simulink model "Test_Model_HR12_2016"  (R2016b)
settings: Solver=FixedStepAuto  StartTime=0.0  StopTime=length(ipoint)  FixedStep=dt  RelTol=1e-3
values from neighbouring files (symbols this model uses):
  Cbx_cyl_fill_efy_intk_mfld_prs_atm_prs_cor_cho = true    [Calib_mdl_RSA.m]
  Cbx_cyl_fill_efy_opt_cho = false    [Calib_mdl_RSA.m]
  Cbx_cyl_fill_igr_opt_cho = false    [Calib_mdl_RSA.m]
  Cbx_ex_vvt_conf = true    [Calib_mdl_RSA.m]
  Cnx_cyl_fill_ex_mfld_prs_cor_cho = 0    [Cal_basic.m]
  Cnx_cyl_nr_conf = 3    [Cal_basic.m]
  Cxx_cyl_fill_efy_drv_max = 20    [Calib_mdl_RSA.m]
  Cxx_cyl_fill_efy_dyn_max = 0.15    [Calib_mdl_RSA.m]
  Cxx_cyl_fill_efy_dyn_min = 0    [Calib_mdl_RSA.m]
  Cxx_cyl_fill_efy_dz = 0.45    [Calib_mdl_RSA.m]
  Cxx_cyl_fill_efy_ovlp_angl = 66    [Calib_mdl_RSA.m]
  Cxx_cyl_fill_efy_vvt_ofs = 0    [Calib_mdl_RSA.m]
  Cxx_cyl_fill_trap_area_h_thd = 0.2    [Cal_basic.m]
  Cxx_cyl_fill_trap_area_l_thd = 0.1    [Cal_basic.m]
  Cxx_cyl_fill_trap_efy_dz_l_thd = 1    [Cal_basic.m]
  Cxx_cyl_fill_trap_efy_dz_neg_slop = -0.5    [Cal_basic.m]
  Cxx_cyl_fill_trap_efy_dz_pos_slop = 0.5    [Cal_basic.m]
  Cxx_cyl_fill_trap_vvt_ovlp_angl = 120    [Calib_mdl_RSA.m]
  Cxx_cyl_vol = 3.9961e-04*3    (= 0.00119883)    [Cal_basic.m]    (also in Calib_mdl_RSA.m = 0.00119900004938)
  Cxx_min_cyl_fill_mdl_ex_mfld_prs_rat_cor = 0    [Cal_basic.m]
  Nnx_eng_run_stt = 2    [Calib_mdl_RSA.m]
  Nxx_atm_kpa = 101.3    [Cal_basic.m]
  Nxx_k_degc = 273.15    [Cal_basic.m]
  Nxx_kilo_bas = 1000    [Cal_basic.m]
  Nxx_wht_pgc_j_kg = 287    [Cal_basic.m]
undefined symbols (not defined in the file or in its folder): Cxx_egr_spc_heat, Cxx_thr_spc_heat, docblock, MapFilling_Aspirated
libraries: AEMS_Standard_Library x78, simulink x2
(part 4 of 5)

== system Test_Model_HR12_2016/ASXX_MWIN_FLW_G/ASXX_MWIN_FLW_G/ASXX_MWIN_FLW_trapexxxxg/ASXX_MWIN_FLW_trapexxxxg_10ms/Trapexxxxg/B2_crossing_angle_correction ==
  Vxx_avg_eng_spd : Inport  Interpolate=off
  Vxx_cyl_fill_efy_intk_mfld_prs_atm_prs_cor : Inport  Port=2  Interpolate=off
  Vxx_vvt_intk_angl : Inport  Port=3  Interpolate=off
  Vxx_vvt_ex_angl : Inport  Port=4  Interpolate=off
  AEMS_Carto_2D_v01_02 : AEMS_Standard_Library/LOOKUP_TABLES/AEMS_LUT_2D  Tag=[LIB]  map_x=Cxb_cyl_fill_eng_spd  map_y=Cxb_cyl_fill_intk_mfld_prs  carto=Cxm_cyl_fill_trap_efy_vvt_ovlp_angl_cor_fac_1
      settings: AttributesFormatString=%<MaskType>\nBkPX=%<map_x>\nBkPY=%<map_y>\nMAP=%<carto>
  AEMS_Carto_2D_v01_1 : AEMS_Standard_Library/LOOKUP_TABLES/AEMS_LUT_2D  Tag=[LIB]  map_x=Cxb_cyl_fill_eng_spd  map_y=Cxb_cyl_fill_intk_mfld_prs  carto=Cxm_cyl_fill_trap_efy_vvt_ovlp_angl_cor_fac_2
      settings: AttributesFormatString=%<MaskType>\nBkPX=%<map_x>\nBkPY=%<map_y>\nMAP=%<carto>
  AEMS_Carto_2D_v01_2 : AEMS_Standard_Library/LOOKUP_TABLES/AEMS_LUT_2D  Tag=[LIB]  map_x=Cxb_cyl_fill_eng_spd  map_y=Cxb_cyl_fill_intk_mfld_prs  carto=Cxm_cyl_fill_trap_efy_vvt_ovlp_angl_cor_fac_3
      settings: AttributesFormatString=%<MaskType>\nBkPX=%<map_x>\nBkPY=%<map_y>\nMAP=%<carto>
  Constant4 : Constant  Value=0  OutDataTypeStr=single
  Cxx_cyl_fill_trap_vvt_ovlp_angl : Constant  Value=Cxx_cyl_fill_trap_vvt_ovlp_angl
  DocBlock : Subsystem  mask(DocBlock){ECoderFlag=, DocumentType=RTF}
      mask prompts: ECoderFlag "Simulink:blocks:docblockEmbeddedCoderFlagLabel"; DocumentType "Simulink:blocks:docblockDocTypeLabel"
      mask help: Use this block to save long descriptive text with the model. Double-clicking the block will open an editor.
      mask TypeOptions DocumentType: Text | RTF | HTML
      mask Display:
      | plot([.8 0 0 1 1 .8 .8 1],[1 1 0 0 .8 1 .8 .8]);
      | text(.5,.6,'DOC','horizontalalignment','center');
      | text(.95,.05,get_param(gcb,'DocumentType'),'verticalalignment','bottom','horizontalalignment','right');
  MinMax : MinMax  Function=max  Inputs=2  OutDataTypeStr=Inherit: Inherit via back propagation  RndMeth=Zero  SaturateOnIntegerOverflow=on  InputSameDT=on
  Product1 : Product  Inputs=**  OutDataTypeStr=Inherit: Inherit via back propagation  RndMeth=Zero
  Product{2..4,6} (4 alike) : Product  OutDataTypeStr=Inherit: Inherit via back propagation  RndMeth=Zero
  Saturation : Saturate  UpperLimit=1  LowerLimit=-1  RndMeth=Zero
      settings: AttributesFormatString=<limits=%<UpperLimit>/%<LowerLimit>>
  Sum1 : Sum  Inputs=+-  OutDataTypeStr=Inherit: Inherit via back propagation  RndMeth=Zero  InputSameDT=on
  Sum2 : Sum  OutDataTypeStr=Inherit: Inherit via back propagation  RndMeth=Zero  InputSameDT=on
  Sum3 : Sum  OutDataTypeStr=Inherit: Inherit via back propagation  RndMeth=Zero  InputSameDT=on
  Sum4 : Sum  OutDataTypeStr=Inherit: Inherit via back propagation  RndMeth=Zero  InputSameDT=on
  Vxx_cyl_fill_trap_efy_vvt_ovlp_angl_cor : Outport
  wires:
  Vxx_cyl_fill_efy_intk_mfld_prs_atm_prs_cor/1 -> AEMS_Carto_2D_v01_1/2, AEMS_Carto_2D_v01_2/2, AEMS_Carto_2D_v01_02/2
  AEMS_Carto_2D_v01_02/1 -> Product4/1  "Vxx_cyl_fill_trap_efy_vvt_ovlp_angl_cor_fac_1"
  Saturation/1 -> Vxx_cyl_fill_trap_efy_vvt_ovlp_angl_cor/1  "Vxx_cyl_fill_trap_efy_vvt_ovlp_angl_cor"
  Product1/1 -> Sum4/2
  Product6/1 -> Sum3/2
  Product4/1 -> Sum3/1
  Sum3/1 -> Sum4/1
  AEMS_Carto_2D_v01_2/1 -> Product1/2  "Vxx_cyl_fill_trap_efy_vvt_ovlp_angl_cor_fac_3"
  Vxx_vvt_intk_angl/1 -> Sum2/1
  Vxx_vvt_ex_angl/1 -> Sum2/2
  Cxx_cyl_fill_trap_vvt_ovlp_angl/1 -> Sum1/2
  Sum2/1 -> Sum1/1
  Sum1/1 -> MinMax/1
  Constant4/1 -> MinMax/2
  Product3/1 -> Product4/2
  Sum4/1 -> Saturation/1
  AEMS_Carto_2D_v01_1/1 -> Product6/2  "Vxx_cyl_fill_trap_efy_vvt_ovlp_angl_cor_fac_2"
  MinMax/1 -> Product2/2, Product1/1, Product2/1, Product3/1
  Product2/1 -> Product3/2, Product6/1
  Vxx_avg_eng_spd/1 -> AEMS_Carto_2D_v01_1/1, AEMS_Carto_2D_v01_2/1, AEMS_Carto_2D_v01_02/1

== system Test_Model_HR12_2016/ASXX_MWIN_FLW_G/ASXX_MWIN_FLW_G/ASXX_MWIN_FLW_trapinxxxg/ASXX_MWIN_FLW_trapinxxxg_10ms/DocBlock/EmptySubsystem ==

== system Test_Model_HR12_2016/ASXX_MWIN_FLW_G/ASXX_MWIN_FLW_G/ASXX_MWIN_FLW_trapinxxxg/ASXX_MWIN_FLW_trapinxxxg_10ms/Trapinxxxg/DocBlock ==
  EmptySubsystem : Subsystem

== system Test_Model_HR12_2016/ASXX_MWIN_FLW_G/ASXX_MWIN_FLW_G/ASXX_MWIN_FLW_filupexxxg/ASXX_MWIN_FLW_filupexxxg_10ms/Filupexxxg/B1_ex_parabolic_correction/DocBlock ==
  EmptySubsystem : Subsystem

== system Test_Model_HR12_2016/ASXX_MWIN_FLW_G/ASXX_MWIN_FLW_G/ASXX_MWIN_FLW_filupexxxg/ASXX_MWIN_FLW_filupexxxg_10ms/Filupexxxg/B2_overlap_correction/DocBlock ==
  EmptySubsystem : Subsystem

== system Test_Model_HR12_2016/ASXX_MWIN_FLW_G/ASXX_MWIN_FLW_G/ASXX_MWIN_FLW_filupxxxxg/ASXX_MWIN_FLW_filupxxxxg_10ms/A_Parabolic_model/A1_altimetric_correction/DocBlock ==
  EmptySubsystem : Subsystem

== system Test_Model_HR12_2016/ASXX_MWIN_FLW_G/ASXX_MWIN_FLW_G/ASXX_MWIN_FLW_filupxxxxg/ASXX_MWIN_FLW_filupxxxxg_10ms/A_Parabolic_model/A2_dynamic_fill_efv/A11_dynamic_fill_efv_thermal_correction ==
  Vxx_avg_eng_spd : Inport  Interpolate=off
  Vxx_intk_mfld_prs : Inport  Port=2  Interpolate=off
  Vxx_tq_fuel_typ_rat : Inport  Port=3  Interpolate=off
  Vxx_cyl_fill_efy_dyn_cor_accel_t_cst_bifuel : Inport  Port=4  Interpolate=off
  Vxx_cyl_fill_efy_dyn_cor_decl_t_cst_bifuel : Inport  Port=5  Interpolate=off
  Vbx_aj_accel_decl : Inport  Port=6  Interpolate=off
  Vxx_cyl_fill_efy_dyn_cor_thrml_bifuel : Inport  Port=7  Interpolate=off
  Vxx_atm_prs : Inport  Port=8  Interpolate=off
  Vxx_cyl_fill_efy_dyn_cor_atm_prs_bifuel : Inport  Port=9  Interpolate=off
  A111_Filter_constant : Subsystem
  A112_Thermal_and_Atmosphere_pressure_Correction : Subsystem
  AEMS_FIRST_ORDER_FILTER_RST : AEMS_Standard_Library/FILTER/AEMS_FIRST_ORDER_FILTER_RST  Tag=[LIB]
      settings: AttributesFormatString=%<MaskType>
  AEMS_TAU_TO_FILTER_PARAM1 : AEMS_Standard_Library/FILTER/AEMS_TAU_TO_FILTER_PARAM  Tag=[LIB]  Nxb_fil_para=Nxb_fil_para  Nxp_fil_para=Nxp_fil_para
      settings: AttributesFormatString=|
      | %<MaskType>
      | Breakpoint: %<Nxb_fil_para>
      | Map: %<Nxp_fil_para>
  Constant7 : Constant  Value=0.01
  Saturation4 : Saturate  UpperLimit=1  LowerLimit=-1  RndMeth=Zero
      settings: AttributesFormatString=<limits=%<UpperLimit>/%<LowerLimit>>
  Sum1 : Sum  Inputs=-+  OutDataTypeStr=Inherit: Inherit via back propagation  RndMeth=Zero  InputSameDT=on
  false : Constant  Value=0  OutDataTypeStr=boolean
  Vxx_cyl_fill_efy_dyn_cor_raw : Outport
  wires:
  Vbx_aj_accel_decl/1 -> A111_Filter_constant/6(Vbx_aj_accel_decl)
  Vxx_cyl_fill_efy_dyn_cor_accel_t_cst_bifuel/1 -> A111_Filter_constant/4(Vxx_cyl_fill_efy_dyn_cor_accel_t_cst_bifuel)
  Vxx_cyl_fill_efy_dyn_cor_decl_t_cst_bifuel/1 -> A111_Filter_constant/5(Vxx_cyl_fill_efy_dyn_cor_decl_t_cst_bifuel)
  A111_Filter_constant/1(Vxx_cyl_fill_efy_dyn_cor_t_cst) -> AEMS_TAU_TO_FILTER_PARAM1/1
  Sum1/1 -> Saturation4/1
  false/1 -> AEMS_FIRST_ORDER_FILTER_RST/4
  Constant7/1 -> AEMS_TAU_TO_FILTER_PARAM1/2
  AEMS_TAU_TO_FILTER_PARAM1/1 -> AEMS_FIRST_ORDER_FILTER_RST/1  "Vxx_cyl_fill_efy_dyn_cor_atm_prs_fil_para"
  AEMS_FIRST_ORDER_FILTER_RST/1 -> Sum1/1  "Vxx_cyl_fill_efy_dyn_cor_atm_prs_fil"
  Saturation4/1 -> Vxx_cyl_fill_efy_dyn_cor_raw/1  "Vxx_cyl_fill_efy_dyn_cor_raw"
  A112_Thermal_and_Atmosphere_pressure_Correction/1(Vxx_cyl_fill_efy_dyn_cor_atm_prs_raw) -> AEMS_FIRST_ORDER_FILTER_RST/3, AEMS_FIRST_ORDER_FILTER_RST/2, Sum1/2
  Vxx_cyl_fill_efy_dyn_cor_thrml_bifuel/1 -> A112_Thermal_and_Atmosphere_pressure_Correction/4(Vxx_cyl_fill_efy_dyn_cor_thrml_bifuel)
  Vxx_atm_prs/1 -> A112_Thermal_and_Atmosphere_pressure_Correction/5(Vxx_atm_prs)
  Vxx_cyl_fill_efy_dyn_cor_atm_prs_bifuel/1 -> A112_Thermal_and_Atmosphere_pressure_Correction/6(Vxx_cyl_fill_efy_dyn_cor_atm_prs_bifuel)
  Vxx_intk_mfld_prs/1 -> A111_Filter_constant/2(Vxx_intk_mfld_prs), A112_Thermal_and_Atmosphere_pressure_Correction/2(Vxx_intk_mfld_prs)
  Vxx_avg_eng_spd/1 -> A112_Thermal_and_Atmosphere_pressure_Correction/1(Vxx_avg_eng_spd), A111_Filter_constant/1(Vxx_avg_eng_spd)
  Vxx_tq_fuel_typ_rat/1 -> A111_Filter_constant/3(Vxx_tq_fuel_typ_rat), A112_Thermal_and_Atmosphere_pressure_Correction/3(Vxx_tq_fuel_typ_rat)

== system Test_Model_HR12_2016/ASXX_MWIN_FLW_G/ASXX_MWIN_FLW_G/ASXX_MWIN_FLW_filupxxxxg/ASXX_MWIN_FLW_filupxxxxg_10ms/A_Parabolic_model/A2_dynamic_fill_efv/DocBlock ==
  EmptySubsystem : Subsystem

== system Test_Model_HR12_2016/ASXX_MWIN_FLW_G/ASXX_MWIN_FLW_G/ASXX_MWIN_FLW_filupxxxxg/ASXX_MWIN_FLW_filupxxxxg_10ms/A_Parabolic_model/A3_fil_efv_cylndr_deactivate/DocBlock ==
  EmptySubsystem : Subsystem

== system Test_Model_HR12_2016/ASXX_MWIN_FLW_G/ASXX_MWIN_FLW_G/ASXX_MWIN_FLW_filupxxxxg/ASXX_MWIN_FLW_filupxxxxg_10ms/A_Parabolic_model/A4_adm_parabolic_correction/DocBlock ==
  EmptySubsystem : Subsystem

== system Test_Model_HR12_2016/ASXX_MWIN_FLW_G/ASXX_MWIN_FLW_G/ASXX_MWIN_FLW_filupxxxxg/ASXX_MWIN_FLW_filupxxxxg_10ms/A_Parabolic_model/A5_vlv_air_temp_correction/DocBlock ==
  EmptySubsystem : Subsystem

== system Test_Model_HR12_2016/ASXX_MWIN_FLW_G/ASXX_MWIN_FLW_G/ASXX_MWIN_FLW_filupxxxxg/ASXX_MWIN_FLW_filupxxxxg_10ms/B_Optional_air_filling_estimation/B1_Pumped_mass_caculation/B11_Normalization_factor ==
  Vxx_intk_vlv_temp : Inport  Interpolate=off
  Vxx_ex_mfld_temp : Inport  Port=2  Interpolate=off
  AEMS_PROTECTED_DIVISION : AEMS_Standard_Library/MATH/AEMS_PROTECTED_DIVISION  Tag=[LIB]  out_mode=Default_Output -> Output  tolerance=200
      settings: AttributesFormatString=%<MaskType>\nOutput when |Denominator| < Tolerance = %<out_mode>\nDenominator Tolerance = %<tolerance>
  Calibration_1 : Constant  Value=Nxx_k_degc
  Constant : Constant  OutDataTypeStr=single
  Demux : Demux  Outputs=2
  Mux : Mux  Inputs=2
  Mux1 : Mux  Inputs=2
  Saturation2 : Saturate  UpperLimit=2  LowerLimit=0  RndMeth=Zero
      settings: AttributesFormatString=<limits=%<UpperLimit>/%<LowerLimit>>
  Sum1 : Sum  OutDataTypeStr=Inherit: Inherit via back propagation  RndMeth=Zero  InputSameDT=on
  Vxx_cyl_fill_mdl_mass_cor_fac : Outport
  wires:
  Vxx_intk_vlv_temp/1 -> Mux/1
  Vxx_ex_mfld_temp/1 -> Mux/2
  AEMS_PROTECTED_DIVISION/1 -> Saturation2/1
  Calibration_1/1 -> Mux1/2, Mux1/1
  Mux/1 -> Sum1/1
  Sum1/1 -> Demux/1
  Demux/1 -> AEMS_PROTECTED_DIVISION/1
  Demux/2 -> AEMS_PROTECTED_DIVISION/2
  Saturation2/1 -> Vxx_cyl_fill_mdl_mass_cor_fac/1  "Vxx_cyl_fill_mdl_mass_cor_fac"
  Mux1/1 -> Sum1/2
  Constant/1 -> AEMS_PROTECTED_DIVISION/3

== system Test_Model_HR12_2016/ASXX_MWIN_FLW_G/ASXX_MWIN_FLW_G/ASXX_MWIN_FLW_filupxxxxg/ASXX_MWIN_FLW_filupxxxxg_10ms/B_Optional_air_filling_estimation/B1_Pumped_mass_caculation/B12_Exhaust_pressure_correction ==
  Vxx_atm_prs : Inport  Interpolate=off
  Vxx_pft_rel_diff_prs : Inport  Port=2  Interpolate=off
  Vxx_ex_mfld_prs : Inport  Port=3  Interpolate=off
  Vxx_mdl_ref_ex_mfld_prs : Inport  Port=4  Interpolate=off
  Vxx_intk_mfld_prs : Inport  Port=5  Interpolate=off
  Vxx_avg_eng_spd : Inport  Port=6  Interpolate=off
  B121_Intk_mfld_prs_diff : Subsystem
  B122_Ex_mfld_prs_cor_fac : Subsystem
  DocBlock : Subsystem  InitFcn=docblock('save_document',gcb);  mask(DocBlock){ECoderFlag=, DocumentType=RTF}
      mask prompts: ECoderFlag "Simulink:masks:DocBlockEmbeddedCoderFlagLabel_MP"; DocumentType "Simulink:masks:DocBlockDocTypeLabel_MP"
      mask help: Simulink:masks:DocBlock_MD
      settings: DeleteFcn=docblock('close_document',gcb);  PreSaveFcn=docblock('save_document',gcb);  OpenFcn=docblock('edit_document',gcb);
      mask TypeOptions DocumentType: Simulink:masks:Text | Simulink:masks:RTF | Simulink:masks:HTML
      mask Display:
      | plot([.8 0 0 1 1 .8 .8 1],[1 1 0 0 .8 1 .8 .8]);
      | text(.5,.6,'DOC','horizontalalignment','center');
      | text(.95,.05,get_param(gcb,'DocumentType'),'verticalalignment','bottom','horizontalalignment','right');
  Vxx_cyl_fill_mdl_intk_mfld_prs_diff_cor : Outport
  Vxx_cyl_fill_mdl_ex_mfld_prs_rat_cor : Outport  Port=2
  Vxx_cyl_fill_mdl_intk_mfld_prs_cor : Outport  Port=3
  wires:
  Vxx_atm_prs/1 -> B122_Ex_mfld_prs_cor_fac/1(Vxx_atm_prs), B121_Intk_mfld_prs_diff/1(Vxx_atm_prs)
  Vxx_ex_mfld_prs/1 -> B122_Ex_mfld_prs_cor_fac/3(Vxx_ex_mfld_prs), B121_Intk_mfld_prs_diff/3(Vxx_ex_mfld_prs)
  Vxx_mdl_ref_ex_mfld_prs/1 -> B122_Ex_mfld_prs_cor_fac/4(Vxx_mdl_ref_ex_mfld_prs), B121_Intk_mfld_prs_diff/4(Vxx_mdl_ref_ex_mfld_prs)
  Vxx_pft_rel_diff_prs/1 -> B122_Ex_mfld_prs_cor_fac/2(Vxx_pft_rel_diff_prs), B121_Intk_mfld_prs_diff/2(Vxx_pft_rel_diff_prs)
  B121_Intk_mfld_prs_diff/1(Vxx_cyl_fill_mdl_intk_mfld_prs_diff_cor) -> Vxx_cyl_fill_mdl_intk_mfld_prs_diff_cor/1
  B122_Ex_mfld_prs_cor_fac/1(Vxx_cyl_fill_mdl_ex_mfld_prs_rat_cor) -> Vxx_cyl_fill_mdl_ex_mfld_prs_rat_cor/1
  Vxx_intk_mfld_prs/1 -> B121_Intk_mfld_prs_diff/5(Vxx_intk_mfld_prs)
  Vxx_avg_eng_spd/1 -> B122_Ex_mfld_prs_cor_fac/6(Vxx_avg_eng_spd), B121_Intk_mfld_prs_diff/6(Vxx_avg_eng_spd)
  B121_Intk_mfld_prs_diff/2(Vxx_cyl_fill_mdl_intk_mfld_prs_cor) -> B122_Ex_mfld_prs_cor_fac/5(Vxx_cyl_fill_mdl_intk_mfld_prs_cor), Vxx_cyl_fill_mdl_intk_mfld_prs_cor/1

== system Test_Model_HR12_2016/ASXX_MWIN_FLW_G/ASXX_MWIN_FLW_G/ASXX_MWIN_FLW_filupxxxxg/ASXX_MWIN_FLW_filupxxxxg_10ms/B_Optional_air_filling_estimation/B1_Pumped_mass_caculation/B13_In_cylinder_ivc_mass ==
  Vxx_intk_vlv_temp : Inport  Interpolate=off
  Vxx_avg_eng_spd : Inport  Port=2  Interpolate=off
  Vxx_intk_mfld_prs : Inport  Port=3  Interpolate=off
  Vxx_vvt_intk_angl_cls : Inport  Port=4  Interpolate=off
  Vxx_vvt_intk_angl_cls_l_lift : Inport  Port=5  Interpolate=off
  AEMS_LUT_1D : AEMS_Standard_Library/LOOKUP_TABLES/AEMS_LUT_1D  Tag=[LIB]  map_x=Cxb_cyl_fill_eng_spd  map_z=Cxp_cyl_fill_mdl_intk_vlv_cls_angl_cor
      settings: AttributesFormatString=%<MaskType>\nBkPX=%<map_x>\nLUT=%<map_z>
  AEMS_LUT_1D1 : AEMS_Standard_Library/LOOKUP_TABLES/AEMS_LUT_1D  Tag=[LIB]  map_x=Cxb_cyl_fill_mdl_intk_vlv_cls_angl_cyl_vol  map_z=Cxp_cyl_fill_mdl_intk_vlv_cls_angl_cyl_vol
      settings: AttributesFormatString=%<MaskType>\nBkPX=%<map_x>\nLUT=%<map_z>
  AEMS_LUT_1D3 : AEMS_Standard_Library/LOOKUP_TABLES/AEMS_LUT_1D  Tag=[LIB]  map_x=Cxb_cyl_fill_eng_spd  map_z=Cxp_cyl_fill_mdl_intk_vlv_cls_angl_cor_vvl_intk_l_lift
      settings: AttributesFormatString=%<MaskType>\nBkPX=%<map_x>\nLUT=%<map_z>
  AEMS_LUT_2D2 : AEMS_Standard_Library/LOOKUP_TABLES/AEMS_LUT_2D  Tag=[LIB]  map_x=Cxb_cyl_fill_eng_spd  map_y=Cxb_cyl_fill_intk_mfld_prs  carto=Cxm_cyl_fill_mdl_cor_1
      settings: AttributesFormatString=%<MaskType>\nBkPX=%<map_x>\nBkPY=%<map_y>\nMAP=%<carto>
  AEMS_LUT_2D7 : AEMS_Standard_Library/LOOKUP_TABLES/AEMS_LUT_2D  Tag=[LIB]  map_x=Cxb_cyl_fill_eng_spd  map_y=Cxb_cyl_fill_intk_mfld_prs  carto=Cxm_cyl_fill_mdl_cor_1_vvl_intk_l_lift
      settings: AttributesFormatString=%<MaskType>\nBkPX=%<map_x>\nBkPY=%<map_y>\nMAP=%<carto>
  AEMS_PROTECTED_DIVISION : AEMS_Standard_Library/MATH/AEMS_PROTECTED_DIVISION  Tag=[LIB]  out_mode=Numerator / Tolerance -> Output  tolerance=57400
      settings: AttributesFormatString=%<MaskType>\nOutput when |Denominator| < Tolerance = %<out_mode>\nDenominator Tolerance = %<tolerance>
  Calibration2 : Constant  Value=1e+6  OutDataTypeStr=single
  Calibration_1 : Constant  Value=Nxx_k_degc
  Mux1 : Mux  Inputs=2
  Mux2 : Mux  Inputs=2
  Mux3 : Mux  Inputs=2
  Nxx_k_degc2 : Constant  Value=Nxx_kilo_bas
  Nxx_wht_pgc2 : Constant  Value=Nxx_wht_pgc_j_kg
  Product{3..5,10,12} (5 alike) : Product  Inputs=**  OutDataTypeStr=Inherit: Inherit via back propagation  RndMeth=Zero
  Saturation1 : Saturate  UpperLimit=5000  LowerLimit=0  RndMeth=Zero
      settings: AttributesFormatString=<limits=%<UpperLimit>/%<LowerLimit>>
  Saturation2 : Saturate  UpperLimit=720  LowerLimit=-60  RndMeth=Zero
      settings: AttributesFormatString=<limits=%<UpperLimit>/%<LowerLimit>>
  Sum1 : Sum  OutDataTypeStr=Inherit: Inherit via back propagation  RndMeth=Zero  InputSameDT=on
  Sum5 : Sum  Inputs=-+  OutDataTypeStr=Inherit: Inherit via back propagation  RndMeth=Zero  InputSameDT=on
  To Workspace4 : ToWorkspace  VariableName=Mivc_bas  SampleTime=1
  Vxt_cyl_fill_mdl_tot_mass_bas_gas : Outport
  wires:
  Product10/1 -> Product4/2
  Nxx_wht_pgc2/1 -> Product3/2
  AEMS_PROTECTED_DIVISION/1 -> Product5/1
  Mux1/1 -> Sum5/2
  Product4/1 -> AEMS_PROTECTED_DIVISION/1
  Sum1/1 -> Product3/1
  Calibration_1/1 -> Sum1/2
  Sum5/1 -> Saturation2/1
  AEMS_LUT_1D/1 -> Mux2/1
  Nxx_k_degc2/1 -> Product10/2
  Product3/1 -> AEMS_PROTECTED_DIVISION/2
  Vxx_avg_eng_spd/1 -> AEMS_LUT_2D7/1, AEMS_LUT_2D2/1, AEMS_LUT_1D/1, AEMS_LUT_1D3/1
  AEMS_LUT_1D1/1 -> Product4/1
  Vxx_intk_mfld_prs/1 -> AEMS_LUT_2D7/2, AEMS_LUT_2D2/2, Product10/1
  AEMS_LUT_2D7/1 -> Mux3/2
  AEMS_LUT_2D2/1 -> Mux3/1
  Mux2/1 -> Sum5/1
  AEMS_LUT_1D3/1 -> Mux2/2
  Mux3/1 -> Product5/2
  Vxx_intk_vlv_temp/1 -> Sum1/1
  Saturation1/1 -> To Workspace4/1, Vxt_cyl_fill_mdl_tot_mass_bas_gas/1  "Vxt_cyl_fill_mdl_tot_mass_bas_gas"
  Calibration2/1 -> Product12/1
  Product5/1 -> Product12/2
  Vxx_vvt_intk_angl_cls/1 -> Mux1/1
  Vxx_vvt_intk_angl_cls_l_lift/1 -> Mux1/2
  Product12/1 -> Saturation1/1
  Saturation2/1 -> AEMS_LUT_1D1/1  "Vxt_vvt_intk_angl_cls_cor"

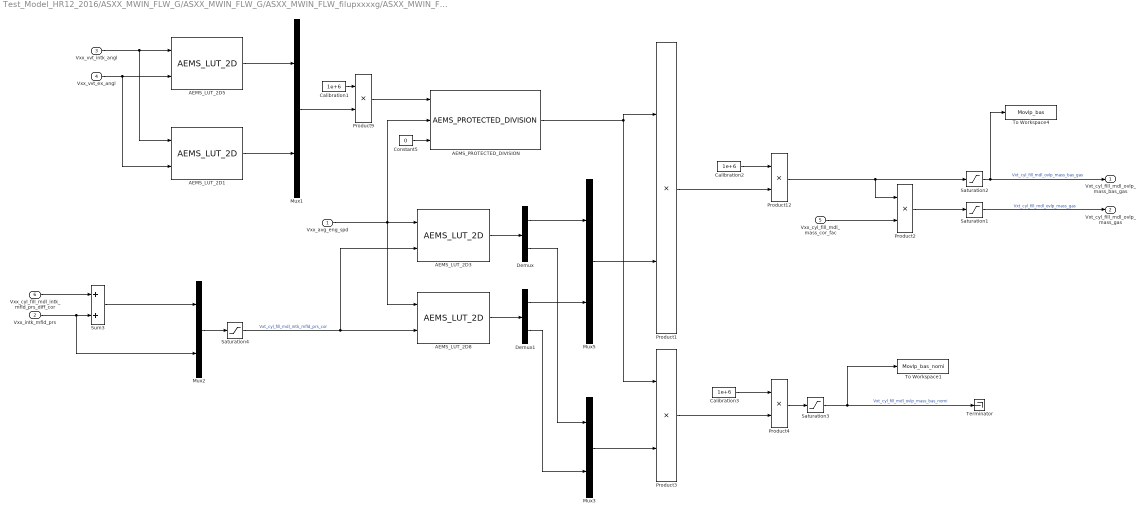
== system Test_Model_HR12_2016/ASXX_MWIN_FLW_G/ASXX_MWIN_FLW_G/ASXX_MWIN_FLW_filupxxxxg/ASXX_MWIN_FLW_filupxxxxg_10ms/B_Optional_air_filling_estimation/B1_Pumped_mass_caculation/B14_In_cylinder_overlap_mass ==
  Vxx_avg_eng_spd : Inport  Interpolate=off
  Vxx_intk_mfld_prs : Inport  Port=2  Interpolate=off
  Vxx_vvt_intk_angl : Inport  Port=3  Interpolate=off
  Vxx_vvt_ex_angl : Inport  Port=4  Interpolate=off
  Vxx_cyl_fill_mdl_mass_cor_fac : Inport  Port=5  Interpolate=off
  Vxx_cyl_fill_mdl_intk_mfld_prs_diff_cor : Inport  Port=6  Interpolate=off
  AEMS_LUT_2D1 : AEMS_Standard_Library/LOOKUP_TABLES/AEMS_LUT_2D  Tag=[LIB]  map_x=Cxb_cyl_fill_mdl_vvt_intk_angl_ovlp_fac  map_y=Cxb_cyl_fill_mdl_vvt_ex_angl_ovlp_fac  carto=Cxm_cyl_fill_mdl_vvt_intk_ex_angl_ovlp_fac_vvl_intk_l_lift
      settings: AttributesFormatString=%<MaskType>\nBkPX=%<map_x>\nBkPY=%<map_y>\nMAP=%<carto>
  AEMS_LUT_2D3 : AEMS_Standard_Library/LOOKUP_TABLES/AEMS_LUT_2D  Tag=[LIB]  map_x=Cxb_cyl_fill_eng_spd  map_y=Cxb_cyl_fill_intk_mfld_prs  carto=Cxm_cyl_fill_mdl_cor_2
      settings: AttributesFormatString=%<MaskType>\nBkPX=%<map_x>\nBkPY=%<map_y>\nMAP=%<carto>
  AEMS_LUT_2D5 : AEMS_Standard_Library/LOOKUP_TABLES/AEMS_LUT_2D  Tag=[LIB]  map_x=Cxb_cyl_fill_mdl_vvt_intk_angl_ovlp_fac  map_y=Cxb_cyl_fill_mdl_vvt_ex_angl_ovlp_fac  carto=Cxm_cyl_fill_mdl_vvt_intk_ex_angl_ovlp_fac
      settings: AttributesFormatString=%<MaskType>\nBkPX=%<map_x>\nBkPY=%<map_y>\nMAP=%<carto>
  AEMS_LUT_2D8 : AEMS_Standard_Library/LOOKUP_TABLES/AEMS_LUT_2D  Tag=[LIB]  map_x=Cxb_cyl_fill_eng_spd  map_y=Cxb_cyl_fill_intk_mfld_prs  carto=Cxm_cyl_fill_mdl_cor_2_vvl_intk_l_lift
      settings: AttributesFormatString=%<MaskType>\nBkPX=%<map_x>\nBkPY=%<map_y>\nMAP=%<carto>
  AEMS_PROTECTED_DIVISION : AEMS_Standard_Library/MATH/AEMS_PROTECTED_DIVISION  Tag=[LIB]  out_mode=Default_Output -> Output  tolerance=300
      settings: AttributesFormatString=%<MaskType>\nOutput when |Denominator| < Tolerance = %<out_mode>\nDenominator Tolerance = %<tolerance>
  Calibration1 : Constant  Value=1e+6  OutDataTypeStr=single
  Calibration2 : Constant  Value=1e+6  OutDataTypeStr=single
  Calibration3 : Constant  Value=1e+6  OutDataTypeStr=single
  Constant5 : Constant  Value=0  OutDataTypeStr=single
  Demux : Demux  Outputs=2
  Demux1 : Demux  Outputs=2
  Mux{1..3,5} (4 alike) : Mux  Inputs=2
  Product{1..4,9,12} (6 alike) : Product  Inputs=**  OutDataTypeStr=Inherit: Inherit via back propagation  RndMeth=Zero
  Saturation1 : Saturate  UpperLimit=5000  LowerLimit=-5000  RndMeth=Zero
      settings: AttributesFormatString=<limits=%<UpperLimit>/%<LowerLimit>>
  Saturation2 : Saturate  UpperLimit=5000  LowerLimit=-5000  RndMeth=Zero
      settings: AttributesFormatString=<limits=%<UpperLimit>/%<LowerLimit>>
  Saturation3 : Saturate  UpperLimit=5000  LowerLimit=-5000  RndMeth=Zero
      settings: AttributesFormatString=<limits=%<UpperLimit>/%<LowerLimit>>
  Saturation4 : Saturate  UpperLimit=2000  LowerLimit=0  RndMeth=Zero
      settings: AttributesFormatString=<limits=%<UpperLimit>/%<LowerLimit>>
  Sum3 : Sum  OutDataTypeStr=Inherit: Inherit via back propagation  RndMeth=Zero  InputSameDT=on
  Terminator : Terminator
  To Workspace1 : ToWorkspace  VariableName=Movlp_bas_nomi  SampleTime=1
  To Workspace4 : ToWorkspace  VariableName=Movlp_bas  SampleTime=1
  Vxt_cyl_fill_mdl_ovlp_mass_bas_gas : Outport
  Vxt_cyl_fill_mdl_ovlp_mass_gas : Outport  Port=2
  wires:
  Vxx_avg_eng_spd/1 -> AEMS_PROTECTED_DIVISION/2, AEMS_LUT_2D8/1, AEMS_LUT_2D3/1
  Vxx_vvt_ex_angl/1 -> AEMS_LUT_2D1/2, AEMS_LUT_2D5/2
  Vxx_vvt_intk_angl/1 -> AEMS_LUT_2D1/1, AEMS_LUT_2D5/1
  AEMS_LUT_2D5/1 -> Mux1/1
  AEMS_LUT_2D1/1 -> Mux1/2
  Calibration1/1 -> Product9/1
  Mux1/1 -> Product9/2
  Product9/1 -> AEMS_PROTECTED_DIVISION/1
  Saturation1/1 -> Vxt_cyl_fill_mdl_ovlp_mass_gas/1  "Vxt_cyl_fill_mdl_ovlp_mass_gas"
  Calibration2/1 -> Product12/1
  Product1/1 -> Product12/2
  AEMS_PROTECTED_DIVISION/1 -> Product1/1, Product3/1
  Vxx_cyl_fill_mdl_mass_cor_fac/1 -> Product2/2
  Product12/1 -> Saturation2/1, Product2/1
  Saturation2/1 -> To Workspace4/1, Vxt_cyl_fill_mdl_ovlp_mass_bas_gas/1  "Vxt_cyl_fill_mdl_ovlp_mass_bas_gas"
  Product2/1 -> Saturation1/1
  Vxx_intk_mfld_prs/1 -> Mux2/2, Sum3/2
  Vxx_cyl_fill_mdl_intk_mfld_prs_diff_cor/1 -> Sum3/1
  AEMS_LUT_2D3/1 -> Demux/1
  AEMS_LUT_2D8/1 -> Demux1/1
  Demux/1 -> Mux5/1
  Demux1/1 -> Mux5/2
  Demux/2 -> Mux3/1
  Demux1/2 -> Mux3/2
  Mux3/1 -> Product3/2
  Calibration3/1 -> Product4/1
  Product3/1 -> Product4/2
  Product4/1 -> Saturation3/1
  Saturation3/1 -> To Workspace1/1, Terminator/1  "Vxt_cyl_fill_mdl_ovlp_mass_bas_nomi"
  Sum3/1 -> Mux2/1
  Mux2/1 -> Saturation4/1
  Mux5/1 -> Product1/2
  Saturation4/1 -> AEMS_LUT_2D3/2, AEMS_LUT_2D8/2  "Vxt_cyl_fill_mdl_intk_mfld_prs_cor"
  Constant5/1 -> AEMS_PROTECTED_DIVISION/3

== system Test_Model_HR12_2016/ASXX_MWIN_FLW_G/ASXX_MWIN_FLW_G/ASXX_MWIN_FLW_filupxxxxg/ASXX_MWIN_FLW_filupxxxxg_10ms/B_Optional_air_filling_estimation/B1_Pumped_mass_caculation/B15_In_cylinder_evc_mass ==
  Vxx_avg_eng_spd : Inport  Interpolate=off
  Vxx_intk_mfld_prs : Inport  Port=2  Interpolate=off
  Vxx_vvt_ex_angl_cls : Inport  Port=3  Interpolate=off
  Vxx_cyl_fill_mdl_mass_cor_fac : Inport  Port=4  Interpolate=off
  Vxx_cyl_fill_mdl_ex_mfld_prs_rat_cor : Inport  Port=5  Interpolate=off
  AEMS_LUT_1D4 : AEMS_Standard_Library/LOOKUP_TABLES/AEMS_LUT_1D  Tag=[LIB]  map_x=Cxb_cyl_fill_mdl_ex_vlv_cls_angl_cyl_vol  map_z=Cxp_cyl_fill_mdl_ex_vlv_cls_angl_cyl_vol
      settings: AttributesFormatString=%<MaskType>\nBkPX=%<map_x>\nLUT=%<map_z>
  AEMS_LUT_2D4 : AEMS_Standard_Library/LOOKUP_TABLES/AEMS_LUT_2D  Tag=[LIB]  map_x=Cxb_cyl_fill_eng_spd  map_y=Cxb_cyl_fill_intk_mfld_prs  carto=Cxm_cyl_fill_mdl_cor_3
      settings: AttributesFormatString=%<MaskType>\nBkPX=%<map_x>\nBkPY=%<map_y>\nMAP=%<carto>
  AEMS_LUT_2D6 : AEMS_Standard_Library/LOOKUP_TABLES/AEMS_LUT_2D  Tag=[LIB]  map_x=Cxb_cyl_fill_eng_spd  map_y=Cxb_cyl_fill_intk_mfld_prs  carto=Cxm_cyl_fill_mdl_cor_3_vvl_intk_l_lift
      settings: AttributesFormatString=%<MaskType>\nBkPX=%<map_x>\nBkPY=%<map_y>\nMAP=%<carto>
  Calibration2 : Constant  Value=1e+6  OutDataTypeStr=single
  Mux4 : Mux  Inputs=2
  Product{1..3,12} (4 alike) : Product  Inputs=**  OutDataTypeStr=Inherit: Inherit via back propagation  RndMeth=Zero
  Saturation1 : Saturate  UpperLimit=5000  LowerLimit=0  RndMeth=Zero
      settings: AttributesFormatString=<limits=%<UpperLimit>/%<LowerLimit>>
  Saturation2 : Saturate  UpperLimit=5000  LowerLimit=0  RndMeth=Zero
      settings: AttributesFormatString=<limits=%<UpperLimit>/%<LowerLimit>>
  Saturation3 : Saturate  UpperLimit=5000  LowerLimit=0  RndMeth=Zero
      settings: AttributesFormatString=<limits=%<UpperLimit>/%<LowerLimit>>
  To Workspace1 : ToWorkspace  VariableName=Mevc_bas  SampleTime=1
  To Workspace4 : ToWorkspace  VariableName=Mevc_bas_nomi  SampleTime=1
  Vxt_cyl_fill_mdl_ex_vlv_cls_mass_bas_gas : Outport
  Vxt_cyl_fill_mdl_ex_vlv_cls_mass_gas : Outport  Port=2
  wires:
  Vxx_intk_mfld_prs/1 -> AEMS_LUT_2D6/2, AEMS_LUT_2D4/2
  Vxx_avg_eng_spd/1 -> AEMS_LUT_2D6/1, AEMS_LUT_2D4/1
  Vxx_vvt_ex_angl_cls/1 -> AEMS_LUT_1D4/1
  AEMS_LUT_2D4/1 -> Mux4/1
  AEMS_LUT_1D4/1 -> Product2/2
  AEMS_LUT_2D6/1 -> Mux4/2
  Mux4/1 -> Product2/1
  Product1/1 -> Saturation1/1
  Saturation1/1 -> Vxt_cyl_fill_mdl_ex_vlv_cls_mass_gas/1  "Vxt_cyl_fill_mdl_ex_vlv_cls_mass_gas"
  Vxx_cyl_fill_mdl_mass_cor_fac/1 -> Product1/2
  Product12/1 -> Saturation2/1, Product1/1
  Saturation2/1 -> To Workspace1/1, Vxt_cyl_fill_mdl_ex_vlv_cls_mass_bas_gas/1  "Vxt_cyl_fill_mdl_ex_vlv_cls_mass_bas_gas"
  Calibration2/1 -> Product3/2
  Vxx_cyl_fill_mdl_ex_mfld_prs_rat_cor/1 -> Product12/1
  Product2/1 -> Product3/1
  Saturation3/1 -> To Workspace4/1, Product12/2  "Vxt_cyl_fill_mdl_ex_vlv_cls_mass_bas_nomi"
  Product3/1 -> Saturation3/1

== system Test_Model_HR12_2016/ASXX_MWIN_FLW_G/ASXX_MWIN_FLW_G/ASXX_MWIN_FLW_filupxxxxg/ASXX_MWIN_FLW_filupxxxxg_10ms/B_Optional_air_filling_estimation/B1_Pumped_mass_caculation/B16_Thermal_corection ==
  Vxt_cyl_fill_mdl_pump_mass_bas : Inport  Interpolate=off
  Vxx_cyl_fill_efy_dyn_cor : Inport  Port=2  Interpolate=off
  Vxx_cyl_fill_efy_temp_cor : Inport  Port=3  Interpolate=off
  Calibration_3 : Constant
  DocBlock : Subsystem  InitFcn=docblock('save_document',gcb);  mask(DocBlock){ECoderFlag=, DocumentType=RTF}
      mask prompts: ECoderFlag "Simulink:masks:DocBlockEmbeddedCoderFlagLabel_MP"; DocumentType "Simulink:masks:DocBlockDocTypeLabel_MP"
      mask help: Simulink:masks:DocBlock_MD
      settings: DeleteFcn=docblock('close_document',gcb);  PreSaveFcn=docblock('save_document',gcb);  OpenFcn=docblock('edit_document',gcb);
      mask TypeOptions DocumentType: Simulink:masks:Text | Simulink:masks:RTF | Simulink:masks:HTML
      mask Display:
      | plot([.8 0 0 1 1 .8 .8 1],[1 1 0 0 .8 1 .8 .8]);
      | text(.5,.6,'DOC','horizontalalignment','center');
      | text(.95,.05,get_param(gcb,'DocumentType'),'verticalalignment','bottom','horizontalalignment','right');
  Product1 : Product  Inputs=**  OutDataTypeStr=Inherit: Inherit via back propagation  RndMeth=Zero
  Product2 : Product  Inputs=**  OutDataTypeStr=Inherit: Inherit via back propagation  RndMeth=Zero
  Saturation2 : Saturate  UpperLimit=5000  LowerLimit=0  RndMeth=Zero
      settings: AttributesFormatString=<limits=%<UpperLimit>/%<LowerLimit>>
  Sum5 : Sum  OutDataTypeStr=Inherit: Inherit via back propagation  RndMeth=Zero  InputSameDT=on
  Vxt_cyl_fill_mdl_pump_mass : Outport
  wires:
  Vxt_cyl_fill_mdl_pump_mass_bas/1 -> Product1/1
  Vxx_cyl_fill_efy_dyn_cor/1 -> Sum5/1
  Vxx_cyl_fill_efy_temp_cor/1 -> Product2/2
  Product1/1 -> Product2/1
  Product2/1 -> Saturation2/1
  Saturation2/1 -> Vxt_cyl_fill_mdl_pump_mass/1  "Vxt_cyl_fill_mdl_pump_mass"
  Calibration_3/1 -> Sum5/2
  Sum5/1 -> Product1/2

== system Test_Model_HR12_2016/ASXX_MWIN_FLW_G/ASXX_MWIN_FLW_G/ASXX_MWIN_FLW_filupxxxxg/ASXX_MWIN_FLW_filupxxxxg_10ms/B_Optional_air_filling_estimation/B1_Pumped_mass_caculation/DocBlock ==
  EmptySubsystem : Subsystem

== system Test_Model_HR12_2016/ASXX_MWIN_FLW_G/ASXX_MWIN_FLW_G/ASXX_MWIN_FLW_filupxxxxg/ASXX_MWIN_FLW_filupxxxxg_10ms/B_Optional_air_filling_estimation/B3_Optional_cylinder_trapping_efficiency/B31_Trapping_Area ==
  Vxx_avg_eng_spd : Inport  Interpolate=off
  Vxx_cyl_fill_mdl_intk_mfld_prs_cor : Inport  Port=2  Interpolate=off
  Vxx_vvt_intk_angl : Inport  Port=3  Interpolate=off
  Vxx_vvt_ex_angl : Inport  Port=4  Interpolate=off
  Vxt_cyl_fill_trap_efy_opt_raw : Inport  Port=5  Interpolate=off
  AEMS_HYST_LEFTRIGHT : AEMS_Standard_Library/HYSTERESIS/AEMS_HYST_LEFTRIGHT  Tag=[LIB]  init=false  Th1_Strict=off  Th2_Strict=off
      settings: AttributesFormatString=%<MaskType>\nOutput false when Input falls to Threshold 1: %<Th1_Strict>\nOutput true when Input increases to Threshold 2: %<Th2_Strict>\nInitial Value = %<init>
  AEMS_LUT_2D1 : AEMS_Standard_Library/LOOKUP_TABLES/AEMS_LUT_2D  Tag=[LIB]  map_x=Cxb_cyl_fill_trap_area_vvt_intk  map_y=Cxb_cyl_fill_trap_area_vvt_ex  carto=Cxm_cyl_fill_trap_area_vvt_intk_vvt_ex
      settings: AttributesFormatString=%<MaskType>\nBkPX=%<map_x>\nBkPY=%<map_y>\nMAP=%<carto>
  AEMS_LUT_2D2 : AEMS_Standard_Library/LOOKUP_TABLES/AEMS_LUT_2D  Tag=[LIB]  map_x=Cxb_cyl_fill_eng_spd  map_y=Cxb_cyl_fill_intk_mfld_prs  carto=Cxm_cyl_fill_trap_area_eng_spd_intk_mfld_prs
      settings: AttributesFormatString=%<MaskType>\nBkPX=%<map_x>\nBkPY=%<map_y>\nMAP=%<carto>
  AEMS_LUT_2D3 : AEMS_Standard_Library/LOOKUP_TABLES/AEMS_LUT_2D  Tag=[LIB]  map_x=Cxb_cyl_fill_trap_area_vvt_intk  map_y=Cxb_cyl_fill_trap_area_vvt_ex  carto=Cxm_cyl_fill_trap_area_vvt_intk_vvt_ex_l_lift
      settings: AttributesFormatString=%<MaskType>\nBkPX=%<map_x>\nBkPY=%<map_y>\nMAP=%<carto>
  Calibration_7 : Constant  Value=Cxx_cyl_fill_trap_area_l_thd
  Calibration_8 : Constant  Value=Cxx_cyl_fill_trap_area_h_thd
  Cxx_cyl_fill_efy_dz : Constant  Value=Cxx_cyl_fill_trap_efy_dz_l_thd
  Logical Operator : Logic  OutDataTypeStr=boolean
  Mux : Mux  Inputs=2
  Product12 : Product  Inputs=**  OutDataTypeStr=Inherit: Inherit via back propagation  RndMeth=Zero
  RelationalOperator2 : RelationalOperator  Operator=<  OutDataTypeStr=boolean  RndMeth=Nearest  InputSameDT=on
  Vbt_cyl_fill_trap_area : Outport
  wires:
  Cxx_cyl_fill_efy_dz/1 -> RelationalOperator2/2
  Logical Operator/1 -> Vbt_cyl_fill_trap_area/1  "Vbt_cyl_fill_trap_area"
  Calibration_8/1 -> AEMS_HYST_LEFTRIGHT/3
  Vxx_avg_eng_spd/1 -> AEMS_LUT_2D2/1
  Product12/1 -> AEMS_HYST_LEFTRIGHT/1  "Vxt_cyl_fill_trap_area"
  Calibration_7/1 -> AEMS_HYST_LEFTRIGHT/2
  RelationalOperator2/1 -> Logical Operator/2
  AEMS_LUT_2D2/1 -> Product12/1
  AEMS_HYST_LEFTRIGHT/1 -> Logical Operator/1
  Vxx_cyl_fill_mdl_intk_mfld_prs_cor/1 -> AEMS_LUT_2D2/2
  Vxx_vvt_ex_angl/1 -> AEMS_LUT_2D3/2, AEMS_LUT_2D1/2
  Vxt_cyl_fill_trap_efy_opt_raw/1 -> RelationalOperator2/1
  AEMS_LUT_2D1/1 -> Mux/1
  Vxx_vvt_intk_angl/1 -> AEMS_LUT_2D3/1, AEMS_LUT_2D1/1
  Mux/1 -> Product12/2
  AEMS_LUT_2D3/1 -> Mux/2

== system Test_Model_HR12_2016/ASXX_MWIN_FLW_G/ASXX_MWIN_FLW_G/ASXX_MWIN_FLW_filupxxxxg/ASXX_MWIN_FLW_filupxxxxg_10ms/B_Optional_air_filling_estimation/B3_Optional_cylinder_trapping_efficiency/DocBlock ==
  EmptySubsystem : Subsystem

== system Test_Model_HR12_2016/ASXX_MWIN_FLW_G/ASXX_MWIN_FLW_G/ASXX_MWIN_FLW_filupxxxxg/ASXX_MWIN_FLW_filupxxxxg_10ms/C_consolidation/C1_filter_for_throttle_command/DocBlock ==
  EmptySubsystem : Subsystem

== system Test_Model_HR12_2016/ASXX_MWIN_FLW_G/ASXX_MWIN_FLW_G/ASXX_MWIN_FLW_trapexxxxg/ASXX_MWIN_FLW_trapexxxxg_10ms/Trapexxxxg/B1_crossing_position_correction/DocBlock ==
  EmptySubsystem : Subsystem

== system Test_Model_HR12_2016/ASXX_MWIN_FLW_G/ASXX_MWIN_FLW_G/ASXX_MWIN_FLW_trapexxxxg/ASXX_MWIN_FLW_trapexxxxg_10ms/Trapexxxxg/B2_crossing_angle_correction/DocBlock ==
  EmptySubsystem : Subsystem

== system Test_Model_HR12_2016/ASXX_MWIN_FLW_G/ASXX_MWIN_FLW_G/ASXX_MWIN_FLW_trapinxxxg/ASXX_MWIN_FLW_trapinxxxg_10ms/Trapinxxxg/DocBlock/EmptySubsystem ==

== system Test_Model_HR12_2016/ASXX_MWIN_FLW_G/ASXX_MWIN_FLW_G/ASXX_MWIN_FLW_filupexxxg/ASXX_MWIN_FLW_filupexxxg_10ms/Filupexxxg/B1_ex_parabolic_correction/DocBlock/EmptySubsystem ==

== system Test_Model_HR12_2016/ASXX_MWIN_FLW_G/ASXX_MWIN_FLW_G/ASXX_MWIN_FLW_filupexxxg/ASXX_MWIN_FLW_filupexxxg_10ms/Filupexxxg/B2_overlap_correction/DocBlock/EmptySubsystem ==

== system Test_Model_HR12_2016/ASXX_MWIN_FLW_G/ASXX_MWIN_FLW_G/ASXX_MWIN_FLW_filupxxxxg/ASXX_MWIN_FLW_filupxxxxg_10ms/A_Parabolic_model/A1_altimetric_correction/DocBlock/EmptySubsystem ==

== system Test_Model_HR12_2016/ASXX_MWIN_FLW_G/ASXX_MWIN_FLW_G/ASXX_MWIN_FLW_filupxxxxg/ASXX_MWIN_FLW_filupxxxxg_10ms/A_Parabolic_model/A2_dynamic_fill_efv/A11_dynamic_fill_efv_thermal_correction/A111_Filter_constant ==
  Vxx_avg_eng_spd : Inport  Interpolate=off
  Vxx_intk_mfld_prs : Inport  Port=2  Interpolate=off
  Vxx_tq_fuel_typ_rat : Inport  Port=3  Interpolate=off
  Vxx_cyl_fill_efy_dyn_cor_accel_t_cst_bifuel : Inport  Port=4  Interpolate=off
  Vxx_cyl_fill_efy_dyn_cor_decl_t_cst_bifuel : Inport  Port=5  Interpolate=off
  Vbx_aj_accel_decl : Inport  Port=6  Interpolate=off
  AEMS_INTERP1 : AEMS_Standard_Library/LOOKUP_TABLES/AEMS_INTERP  Tag=[LIB]  Description=This library calculates interpolation for 2 inputs.
      settings: AttributesFormatString=%<MaskType>
  AEMS_INTERP2 : AEMS_Standard_Library/LOOKUP_TABLES/AEMS_INTERP  Tag=[LIB]  Description=This library calculates interpolation for 2 inputs.
      settings: AttributesFormatString=%<MaskType>
  Cmp_fill_efy_n_map_decl_ftc1 : AEMS_Standard_Library/LOOKUP_TABLES/AEMS_LUT_2D  Tag=[LIB]  map_x=Cxb_cyl_fill_efy_dyn_cor_eng_spd  map_y=Cxb_cyl_fill_efy_dyn_cor_intk_mfld_prs  carto=Cxm_cyl_fill_efy_dyn_cor_decl_t_cst
      settings: AttributesFormatString=%<MaskType>\nBkPX=%<map_x>\nBkPY=%<map_y>\nMAP=%<carto>
  Cxm_cyl_fill_efy_dyn_cor_accel_t_cst : AEMS_Standard_Library/LOOKUP_TABLES/AEMS_LUT_2D  Tag=[LIB]  map_x=Cxb_cyl_fill_efy_dyn_cor_eng_spd  map_y=Cxb_cyl_fill_efy_dyn_cor_intk_mfld_prs  carto=Cxm_cyl_fill_efy_dyn_cor_accel_t_cst
      settings: AttributesFormatString=%<MaskType>\nBkPX=%<map_x>\nBkPY=%<map_y>\nMAP=%<carto>
  Saturation2 : Saturate  UpperLimit=6.553499755859375e+02  LowerLimit=0  RndMeth=Zero
      settings: AttributesFormatString=<limits=%<UpperLimit>/%<LowerLimit>>
  Saturation3 : Saturate  UpperLimit=6.553499755859375e+02  LowerLimit=0  RndMeth=Zero
      settings: AttributesFormatString=<limits=%<UpperLimit>/%<LowerLimit>>
  Switch1 : Switch  Criteria=u2 ~= 0  RndMeth=Zero  SaturateOnIntegerOverflow=on  InputSameDT=on
      settings: AttributesFormatString=Criteria=%<Criteria>
  Vxx_cyl_fill_efy_dyn_cor_t_cst : Outport
  wires:
  Vxx_cyl_fill_efy_dyn_cor_accel_t_cst_bifuel/1 -> AEMS_INTERP1/1
  Vbx_aj_accel_decl/1 -> Switch1/2
  Vxx_cyl_fill_efy_dyn_cor_decl_t_cst_bifuel/1 -> AEMS_INTERP2/1
  Switch1/1 -> Vxx_cyl_fill_efy_dyn_cor_t_cst/1  "Vxx_cyl_fill_efy_dyn_cor_t_cst"
  AEMS_INTERP2/1 -> Saturation3/1
  Cmp_fill_efy_n_map_decl_ftc1/1 -> AEMS_INTERP2/3
  Vxx_avg_eng_spd/1 -> Cxm_cyl_fill_efy_dyn_cor_accel_t_cst/1, Cmp_fill_efy_n_map_decl_ftc1/1
  Vxx_intk_mfld_prs/1 -> Cmp_fill_efy_n_map_decl_ftc1/2, Cxm_cyl_fill_efy_dyn_cor_accel_t_cst/2
  Vxx_tq_fuel_typ_rat/1 -> AEMS_INTERP2/2, AEMS_INTERP1/2
  Saturation2/1 -> Switch1/1  "Vxx_cyl_fill_efy_dyn_cor_accel_t_cst"
  AEMS_INTERP1/1 -> Saturation2/1
  Cxm_cyl_fill_efy_dyn_cor_accel_t_cst/1 -> AEMS_INTERP1/3
  Saturation3/1 -> Switch1/3  "Vxx_cyl_fill_efy_dyn_cor_decl_t_cst"

== system Test_Model_HR12_2016/ASXX_MWIN_FLW_G/ASXX_MWIN_FLW_G/ASXX_MWIN_FLW_filupxxxxg/ASXX_MWIN_FLW_filupxxxxg_10ms/A_Parabolic_model/A2_dynamic_fill_efv/A11_dynamic_fill_efv_thermal_correction/A112_Thermal_and_Atmosphere_pressure_Correction ==
  Vxx_avg_eng_spd : Inport  Interpolate=off
  Vxx_intk_mfld_prs : Inport  Port=2  Interpolate=off
  Vxx_tq_fuel_typ_rat : Inport  Port=3  Interpolate=off
  Vxx_cyl_fill_efy_dyn_cor_thrml_bifuel : Inport  Port=4  Interpolate=off
  Vxx_atm_prs : Inport  Port=5  Interpolate=off
  Vxx_cyl_fill_efy_dyn_cor_atm_prs_bifuel : Inport  Port=6  Interpolate=off
  AEMS_Carto_1D_v01_02 : AEMS_Standard_Library/LOOKUP_TABLES/AEMS_LUT_1D  Tag=[LIB]  map_x=Cxb_cyl_fill_efy_dyn_cor_atm_prs_rat  map_z=Cxp_cyl_fill_efy_dyn_cor_atm_prs_rat
      settings: AttributesFormatString=%<MaskType>\nBkPX=%<map_x>\nLUT=%<map_z>
  AEMS_Carto_2D_v01_02 : AEMS_Standard_Library/LOOKUP_TABLES/AEMS_LUT_2D  Tag=[LIB]  map_x=Cxb_cyl_fill_eng_spd  map_y=Cxb_cyl_fill_intk_mfld_prs  carto=Cxm_cyl_fill_efy_dyn_cor_atm_prs
      settings: AttributesFormatString=%<MaskType>\nBkPX=%<map_x>\nBkPY=%<map_y>\nMAP=%<carto>
  AEMS_INTERP1 : AEMS_Standard_Library/LOOKUP_TABLES/AEMS_INTERP  Tag=[LIB]  Description=This library calculates interpolation for 2 inputs.
      settings: AttributesFormatString=%<MaskType>
  AEMS_INTERP2 : AEMS_Standard_Library/LOOKUP_TABLES/AEMS_INTERP  Tag=[LIB]  Description=This library calculates interpolation for 2 inputs.
      settings: AttributesFormatString=%<MaskType>
  Constant3 : Constant
  Cxm_cyl_fill_efy_dyn_cor_thrml : AEMS_Standard_Library/LOOKUP_TABLES/AEMS_LUT_2D  Tag=[LIB]  map_x=Cxb_cyl_fill_eng_spd  map_y=Cxb_cyl_fill_intk_mfld_prs  carto=Cxm_cyl_fill_efy_dyn_cor_thrml
      settings: AttributesFormatString=%<MaskType>\nBkPX=%<map_x>\nBkPY=%<map_y>\nMAP=%<carto>
  Product1 : Product  OutDataTypeStr=Inherit: Inherit via back propagation  RndMeth=Zero
  Product2 : Product  OutDataTypeStr=Inherit: Inherit via back propagation  RndMeth=Zero
  Saturation : Saturate  UpperLimit=1  LowerLimit=-1  RndMeth=Zero
      settings: AttributesFormatString=<limits=%<UpperLimit>/%<LowerLimit>>
  Sum2 : Sum  Inputs=+-  OutDataTypeStr=Inherit: Inherit via back propagation  RndMeth=Zero  InputSameDT=on
  Sum3 : Sum  OutDataTypeStr=Inherit: Inherit via back propagation  RndMeth=Zero  InputSameDT=on
  Vxx_cyl_fill_efy_dyn_cor_atm_prs_raw : Outport
  wires:
  Saturation/1 -> Vxx_cyl_fill_efy_dyn_cor_atm_prs_raw/1  "Vxx_cyl_fill_efy_dyn_cor_atm_prs_raw"
  Vxx_atm_prs/1 -> AEMS_Carto_1D_v01_02/1
  Vxx_cyl_fill_efy_dyn_cor_atm_prs_bifuel/1 -> AEMS_INTERP2/1
  Vxx_cyl_fill_efy_dyn_cor_thrml_bifuel/1 -> AEMS_INTERP1/1
  Constant3/1 -> Sum2/1
  Cxm_cyl_fill_efy_dyn_cor_thrml/1 -> AEMS_INTERP1/3
  AEMS_Carto_2D_v01_02/1 -> AEMS_INTERP2/3
  AEMS_INTERP2/1 -> Product2/2
  AEMS_INTERP1/1 -> Product1/1
  Product1/1 -> Sum3/1
  Product2/1 -> Sum3/2
  Sum3/1 -> Saturation/1
  Sum2/1 -> Product1/2
  AEMS_Carto_1D_v01_02/1 -> Sum2/2, Product2/1
  Vxx_intk_mfld_prs/1 -> AEMS_Carto_2D_v01_02/2, Cxm_cyl_fill_efy_dyn_cor_thrml/2
  Vxx_avg_eng_spd/1 -> Cxm_cyl_fill_efy_dyn_cor_thrml/1, AEMS_Carto_2D_v01_02/1
  Vxx_tq_fuel_typ_rat/1 -> AEMS_INTERP2/2, AEMS_INTERP1/2

== system Test_Model_HR12_2016/ASXX_MWIN_FLW_G/ASXX_MWIN_FLW_G/ASXX_MWIN_FLW_filupxxxxg/ASXX_MWIN_FLW_filupxxxxg_10ms/A_Parabolic_model/A2_dynamic_fill_efv/DocBlock/EmptySubsystem ==

== system Test_Model_HR12_2016/ASXX_MWIN_FLW_G/ASXX_MWIN_FLW_G/ASXX_MWIN_FLW_filupxxxxg/ASXX_MWIN_FLW_filupxxxxg_10ms/A_Parabolic_model/A3_fil_efv_cylndr_deactivate/DocBlock/EmptySubsystem ==

== system Test_Model_HR12_2016/ASXX_MWIN_FLW_G/ASXX_MWIN_FLW_G/ASXX_MWIN_FLW_filupxxxxg/ASXX_MWIN_FLW_filupxxxxg_10ms/A_Parabolic_model/A4_adm_parabolic_correction/DocBlock/EmptySubsystem ==

== system Test_Model_HR12_2016/ASXX_MWIN_FLW_G/ASXX_MWIN_FLW_G/ASXX_MWIN_FLW_filupxxxxg/ASXX_MWIN_FLW_filupxxxxg_10ms/A_Parabolic_model/A5_vlv_air_temp_correction/DocBlock/EmptySubsystem ==

== system Test_Model_HR12_2016/ASXX_MWIN_FLW_G/ASXX_MWIN_FLW_G/ASXX_MWIN_FLW_filupxxxxg/ASXX_MWIN_FLW_filupxxxxg_10ms/B_Optional_air_filling_estimation/B1_Pumped_mass_caculation/B12_Exhaust_pressure_correction/B121_Intk_mfld_prs_diff ==
  Vxx_atm_prs : Inport  Interpolate=off
  Vxx_pft_rel_diff_prs : Inport  Port=2  Interpolate=off
  Vxx_ex_mfld_prs : Inport  Port=3  Interpolate=off
  Vxx_mdl_ref_ex_mfld_prs : Inport  Port=4  Interpolate=off
  Vxx_intk_mfld_prs : Inport  Port=5  Interpolate=off
  Vxx_avg_eng_spd : Inport  Port=6  Interpolate=off
  AEMS_LUT_1D1 : AEMS_Standard_Library/LOOKUP_TABLES/AEMS_LUT_1D  Tag=[LIB]  map_x=Cxb_cyl_fill_mdl_intk_mfld_prs_diff_bas  map_z=Cxp_cyl_fill_mdl_intk_mfld_prs_diff
      settings: AttributesFormatString=%<MaskType>\nBkPX=%<map_x>\nLUT=%<map_z>
  AEMS_LUT_2D2 : AEMS_Standard_Library/LOOKUP_TABLES/AEMS_LUT_2D  Tag=[LIB]  map_x=Cxb_cyl_fill_eng_spd  map_y=Cxb_cyl_fill_intk_mfld_prs  carto=Cxm_cyl_fill_mdl_intk_mfld_prs_diff_cor_fac
      settings: AttributesFormatString=%<MaskType>\nBkPX=%<map_x>\nBkPY=%<map_y>\nMAP=%<carto>
  Multiport Switch : MultiPortSwitch  DataPortOrder=Zero-based contiguous
      settings: AttributesFormatString=PortOrder=%<DataPortOrder>
  Nxx_atm_hpa : Constant  Value=Nxx_atm_kpa
  Nxx_atm_hpa1 : Constant  Value=0  OutDataTypeStr=single
  Nxx_wht_pgc2 : Constant  Value=Cnx_cyl_fill_ex_mfld_prs_cor_cho
  Product3 : Product  Inputs=**  OutDataTypeStr=Inherit: Inherit via back propagation  RndMeth=Zero
  Saturation : Saturate  UpperLimit=1000  LowerLimit=-1000
      settings: AttributesFormatString=<limits=%<UpperLimit>/%<LowerLimit>>
  Saturation1 : Saturate  UpperLimit=1000  LowerLimit=-1000
      settings: AttributesFormatString=<limits=%<UpperLimit>/%<LowerLimit>>
  Saturation2 : Saturate  UpperLimit=2000  LowerLimit=0
      settings: AttributesFormatString=<limits=%<UpperLimit>/%<LowerLimit>>
  Sum1 : Sum  OutDataTypeStr=Inherit: Inherit via back propagation  RndMeth=Zero  InputSameDT=on
  Sum2 : Sum  Inputs=+-  OutDataTypeStr=Inherit: Inherit via back propagation  RndMeth=Zero  InputSameDT=on
  Sum3 : Sum  Inputs=+-  OutDataTypeStr=Inherit: Inherit via back propagation  RndMeth=Zero  InputSameDT=on
  Sum4 : Sum  OutDataTypeStr=Inherit: Inherit via back propagation  RndMeth=Zero  InputSameDT=on
  To Workspace4 : ToWorkspace  VariableName=Pexh_diff  SampleTime=1
  Vxx_cyl_fill_mdl_intk_mfld_prs_diff_cor : Outport
  Vxx_cyl_fill_mdl_intk_mfld_prs_cor : Outport  Port=2
  wires:
  Vxx_pft_rel_diff_prs/1 -> Sum4/2
  Nxx_atm_hpa/1 -> Sum2/1
  Vxx_mdl_ref_ex_mfld_prs/1 -> Sum3/1
  Vxx_ex_mfld_prs/1 -> Sum3/2
  Vxx_atm_prs/1 -> Sum4/1
  Nxx_wht_pgc2/1 -> Multiport Switch/1
  Nxx_atm_hpa1/1 -> Multiport Switch/2
  Multiport Switch/1 -> Saturation1/1
  Sum3/1 -> Multiport Switch/3
  Saturation/1 -> Vxx_cyl_fill_mdl_intk_mfld_prs_diff_cor/1  "Vxx_cyl_fill_mdl_intk_mfld_prs_diff_cor"
  Product3/1 -> Saturation/1
  AEMS_LUT_2D2/1 -> Product3/1
  AEMS_LUT_1D1/1 -> To Workspace4/1, Product3/2  "Vxx_cyl_fill_mdl_intk_mfld_prs_diff"
  Vxx_avg_eng_spd/1 -> AEMS_LUT_2D2/1
  Saturation1/1 -> AEMS_LUT_1D1/1  "Vxx_cyl_fill_mdl_intk_mfld_prs_diff_bas"
  Sum4/1 -> Sum2/2
  Sum2/1 -> Sum1/2, Multiport Switch/4
  Vxx_intk_mfld_prs/1 -> Sum1/1
  Sum1/1 -> Saturation2/1
  Saturation2/1 -> Vxx_cyl_fill_mdl_intk_mfld_prs_cor/1, AEMS_LUT_2D2/2  "Vxx_cyl_fill_mdl_intk_mfld_prs_cor"

== system Test_Model_HR12_2016/ASXX_MWIN_FLW_G/ASXX_MWIN_FLW_G/ASXX_MWIN_FLW_filupxxxxg/ASXX_MWIN_FLW_filupxxxxg_10ms/B_Optional_air_filling_estimation/B1_Pumped_mass_caculation/B12_Exhaust_pressure_correction/B122_Ex_mfld_prs_cor_fac ==
  Vxx_atm_prs : Inport  Interpolate=off
  Vxx_pft_rel_diff_prs : Inport  Port=2  Interpolate=off
  Vxx_ex_mfld_prs : Inport  Port=3  Interpolate=off
  Vxx_mdl_ref_ex_mfld_prs : Inport  Port=4  Interpolate=off
  Vxx_cyl_fill_mdl_intk_mfld_prs_cor : Inport  Port=5  Interpolate=off
  Vxx_avg_eng_spd : Inport  Port=6  Interpolate=off
  AEMS_LUT_1D1 : AEMS_Standard_Library/LOOKUP_TABLES/AEMS_LUT_1D  Tag=[LIB]  map_x=Cxb_cyl_fill_mdl_ex_mfld_prs_rat_bas  map_z=Cxp_cyl_fill_mdl_ex_mfld_prs_rat
      settings: AttributesFormatString=%<MaskType>\nBkPX=%<map_x>\nLUT=%<map_z>
  AEMS_LUT_2D2 : AEMS_Standard_Library/LOOKUP_TABLES/AEMS_LUT_2D  Tag=[LIB]  map_x=Cxb_cyl_fill_eng_spd  map_y=Cxb_cyl_fill_intk_mfld_prs  carto=Cxm_cyl_fill_mdl_ex_mfld_prs_rat_cor_fac
      settings: AttributesFormatString=%<MaskType>\nBkPX=%<map_x>\nBkPY=%<map_y>\nMAP=%<carto>
  AEMS_PROTECTED_DIVISION : AEMS_Standard_Library/MATH/AEMS_PROTECTED_DIVISION  Tag=[LIB]  out_mode=Default_Output -> Output  tolerance=0.001
      settings: AttributesFormatString=%<MaskType>\nOutput when |Denominator| < Tolerance = %<out_mode>\nDenominator Tolerance = %<tolerance>
  Divide : Product  Inputs=*/  OutDataTypeStr=Inherit: Inherit via back propagation
  Multiport Switch : MultiPortSwitch  DataPortOrder=Zero-based contiguous
      settings: AttributesFormatString=PortOrder=%<DataPortOrder>
  Nxx_atm_hpa : Constant  Value=Nxx_atm_kpa
  Nxx_atm_hpa{1..4} (4 alike) : Constant  OutDataTypeStr=single
  Nxx_wht_pgc2 : Constant  Value=Cnx_cyl_fill_ex_mfld_prs_cor_cho
  Product3 : Product  Inputs=**  OutDataTypeStr=Inherit: Inherit via back propagation  RndMeth=Zero
  Saturation : Saturate  UpperLimit=10  LowerLimit=Cxx_min_cyl_fill_mdl_ex_mfld_prs_rat_cor
      settings: AttributesFormatString=<limits=%<UpperLimit>/%<LowerLimit>>
  Saturation1 : Saturate  UpperLimit=10  LowerLimit=0
      settings: AttributesFormatString=<limits=%<UpperLimit>/%<LowerLimit>>
  Sum1 : Sum  OutDataTypeStr=Inherit: Inherit via back propagation  RndMeth=Zero  InputSameDT=on
  Sum3 : Sum  Inputs=+-  OutDataTypeStr=Inherit: Inherit via back propagation  RndMeth=Zero  InputSameDT=on
  Sum4 : Sum  OutDataTypeStr=Inherit: Inherit via back propagation  RndMeth=Zero  InputSameDT=on
  To Workspace4 : ToWorkspace  VariableName=Pexh_ratio  SampleTime=1
  Vxx_cyl_fill_mdl_ex_mfld_prs_rat_cor : Outport
  wires:
  Multiport Switch/1 -> Saturation1/1
  Nxx_atm_hpa1/1 -> Multiport Switch/2
  Nxx_wht_pgc2/1 -> Multiport Switch/1
  Vxx_atm_prs/1 -> Sum1/1
  Vxx_ex_mfld_prs/1 -> AEMS_PROTECTED_DIVISION/1
  Vxx_mdl_ref_ex_mfld_prs/1 -> AEMS_PROTECTED_DIVISION/2
  Vxx_pft_rel_diff_prs/1 -> Sum1/2
  AEMS_PROTECTED_DIVISION/1 -> Multiport Switch/3
  Nxx_atm_hpa/1 -> Divide/2
  Divide/1 -> Multiport Switch/4
  Nxx_atm_hpa2/1 -> AEMS_PROTECTED_DIVISION/3
  Saturation/1 -> Vxx_cyl_fill_mdl_ex_mfld_prs_rat_cor/1  "Vxx_cyl_fill_mdl_ex_mfld_prs_rat_cor"
  AEMS_LUT_1D1/1 -> Sum3/1  "Vxx_cyl_fill_mdl_ex_mfld_prs_rat"
  Saturation1/1 -> To Workspace4/1, AEMS_LUT_1D1/1  "Vxx_cyl_fill_mdl_ex_mfld_prs_rat_bas"
  Vxx_avg_eng_spd/1 -> AEMS_LUT_2D2/1
  Sum1/1 -> Divide/1
  Vxx_cyl_fill_mdl_intk_mfld_prs_cor/1 -> AEMS_LUT_2D2/2
  AEMS_LUT_2D2/1 -> Product3/1
  Sum4/1 -> Saturation/1
  Product3/1 -> Sum4/1
  Nxx_atm_hpa3/1 -> Sum4/2
  Nxx_atm_hpa4/1 -> Sum3/2
  Sum3/1 -> Product3/2

== system Test_Model_HR12_2016/ASXX_MWIN_FLW_G/ASXX_MWIN_FLW_G/ASXX_MWIN_FLW_filupxxxxg/ASXX_MWIN_FLW_filupxxxxg_10ms/B_Optional_air_filling_estimation/B1_Pumped_mass_caculation/B12_Exhaust_pressure_correction/DocBlock ==
  EmptySubsystem : Subsystem

== system Test_Model_HR12_2016/ASXX_MWIN_FLW_G/ASXX_MWIN_FLW_G/ASXX_MWIN_FLW_filupxxxxg/ASXX_MWIN_FLW_filupxxxxg_10ms/B_Optional_air_filling_estimation/B1_Pumped_mass_caculation/B16_Thermal_corection/DocBlock ==
  EmptySubsystem : Subsystem

== system Test_Model_HR12_2016/ASXX_MWIN_FLW_G/ASXX_MWIN_FLW_G/ASXX_MWIN_FLW_filupxxxxg/ASXX_MWIN_FLW_filupxxxxg_10ms/B_Optional_air_filling_estimation/B1_Pumped_mass_caculation/DocBlock/EmptySubsystem ==

== system Test_Model_HR12_2016/ASXX_MWIN_FLW_G/ASXX_MWIN_FLW_G/ASXX_MWIN_FLW_filupxxxxg/ASXX_MWIN_FLW_filupxxxxg_10ms/B_Optional_air_filling_estimation/B3_Optional_cylinder_trapping_efficiency/DocBlock/EmptySubsystem ==

== system Test_Model_HR12_2016/ASXX_MWIN_FLW_G/ASXX_MWIN_FLW_G/ASXX_MWIN_FLW_filupxxxxg/ASXX_MWIN_FLW_filupxxxxg_10ms/C_consolidation/C1_filter_for_throttle_command/DocBlock/EmptySubsystem ==

== system Test_Model_HR12_2016/ASXX_MWIN_FLW_G/ASXX_MWIN_FLW_G/ASXX_MWIN_FLW_trapexxxxg/ASXX_MWIN_FLW_trapexxxxg_10ms/Trapexxxxg/B1_crossing_position_correction/DocBlock/EmptySubsystem ==

== system Test_Model_HR12_2016/ASXX_MWIN_FLW_G/ASXX_MWIN_FLW_G/ASXX_MWIN_FLW_trapexxxxg/ASXX_MWIN_FLW_trapexxxxg_10ms/Trapexxxxg/B2_crossing_angle_correction/DocBlock/EmptySubsystem ==

== system Test_Model_HR12_2016/ASXX_MWIN_FLW_G/ASXX_MWIN_FLW_G/ASXX_MWIN_FLW_filupxxxxg/ASXX_MWIN_FLW_filupxxxxg_10ms/B_Optional_air_filling_estimation/B1_Pumped_mass_caculation/B12_Exhaust_pressure_correction/DocBlock/EmptySubsystem ==

== system Test_Model_HR12_2016/ASXX_MWIN_FLW_G/ASXX_MWIN_FLW_G/ASXX_MWIN_FLW_filupxxxxg/ASXX_MWIN_FLW_filupxxxxg_10ms/B_Optional_air_filling_estimation/B1_Pumped_mass_caculation/B16_Thermal_corection/DocBlock/EmptySubsystem ==
